simulink model "AMR_MotorStartupUnit_MoboticDrive_24a"  (R2024a)
settings: configuration reference "SharedConfig" (kept outside this file)
settings Model: DataDictionary=configuration_dictionary.sldd  SimulationMode=external  Creator=matlab.cut  LastModifiedBy=rodri
settings ConfigSetRef: SourceName=SharedConfig

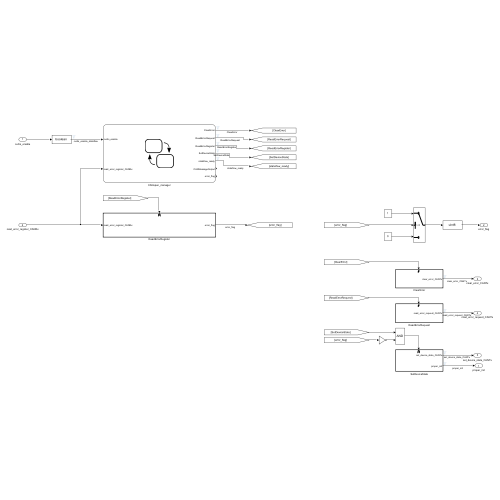
[thumbnail: Simulink's stored preview of the top-level diagram]
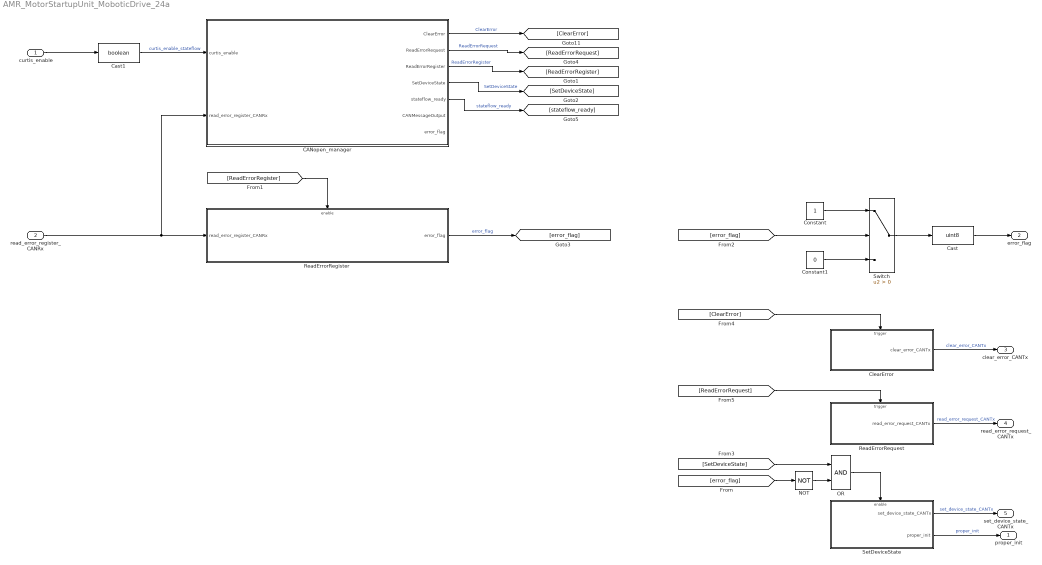
== system AMR_MotorStartupUnit_MoboticDrive_24a ==
  curtis_enable : Inport
  read_error_register_CANRx : Inport  Port=2
  CANopen_manager : Stateflow chart  TreatAsAtomicUnit=on
  Cast : DataTypeConversion  OutDataTypeStr=uint8  SaturateOnIntegerOverflow=off  RndMeth=Floor
  Cast1 : DataTypeConversion  OutDataTypeStr=boolean  SaturateOnIntegerOverflow=off  RndMeth=Floor
  ClearError : Subsystem  TreatAsAtomicUnit=on
  Constant : Constant
  Constant1 : Constant  Value=0
  NOT : Logic  Operator=NOT  IconShape=distinctive  AllPortsSameDT=off  OutDataTypeStr=boolean
  OR : Logic  AllPortsSameDT=off  OutDataTypeStr=boolean
  ReadErrorRegister : Subsystem  TreatAsAtomicUnit=on
  ReadErrorRequest : Subsystem  TreatAsAtomicUnit=on
  SetDeviceState : Subsystem  TreatAsAtomicUnit=on
  Switch : Switch  Criteria=u2 > Threshold  SaturateOnIntegerOverflow=off  InputSameDT=off
  proper_init : Outport
  error_flag : Outport  Port=2
  clear_error_CANTx : Outport  Port=3
  read_error_request_CANTx : Outport  Port=4
  set_device_state_CANTx : Outport  Port=5
  wires:
  [error_flag] -> Switch/2
  Switch/1 -> Cast/1
  Cast/1 -> error_flag/1
  [SetDeviceState] -> OR/1
  [error_flag] -> NOT/1
  curtis_enable/1 -> Cast1/1
  Constant/1 -> Switch/1
  Constant1/1 -> Switch/3
  ReadErrorRegister/1(error_flag) -> [error_flag]  "error_flag"
  NOT/1 -> OR/2
  [ReadErrorRegister] -> ReadErrorRegister/Enable
  ClearError/1(clear_error_CANTx) -> clear_error_CANTx/1  "clear_error_CANTx"
  read_error_register_CANRx/1 -> CANopen_manager/2(read_error_register_CANRx), ReadErrorRegister/1(read_error_register_CANRx)
  SetDeviceState/1(set_device_state_CANTx) -> set_device_state_CANTx/1  "set_device_state_CANTx"
  ReadErrorRequest/1(read_error_request_CANTx) -> read_error_request_CANTx/1  "read_error_request_CANTx"
  SetDeviceState/2(proper_init) -> proper_init/1  "proper_init"
  CANopen_manager/2(ReadErrorRequest) -> [ReadErrorRequest]  "ReadErrorRequest"
  CANopen_manager/5(stateflow_ready) -> [stateflow_ready]  "stateflow_ready"
  Cast1/1 -> CANopen_manager/1(curtis_enable)  "curtis_enable_stateflow"
  CANopen_manager/3(ReadErrorRegister) -> [ReadErrorRegister]  "ReadErrorRegister"
  CANopen_manager/1(ClearError) -> [ClearError]  "ClearError"
  CANopen_manager/4(SetDeviceState) -> [SetDeviceState]  "SetDeviceState"
  OR/1 -> SetDeviceState/Enable
  [ClearError] -> ClearError/Trigger
  [ReadErrorRequest] -> ReadErrorRequest/Trigger

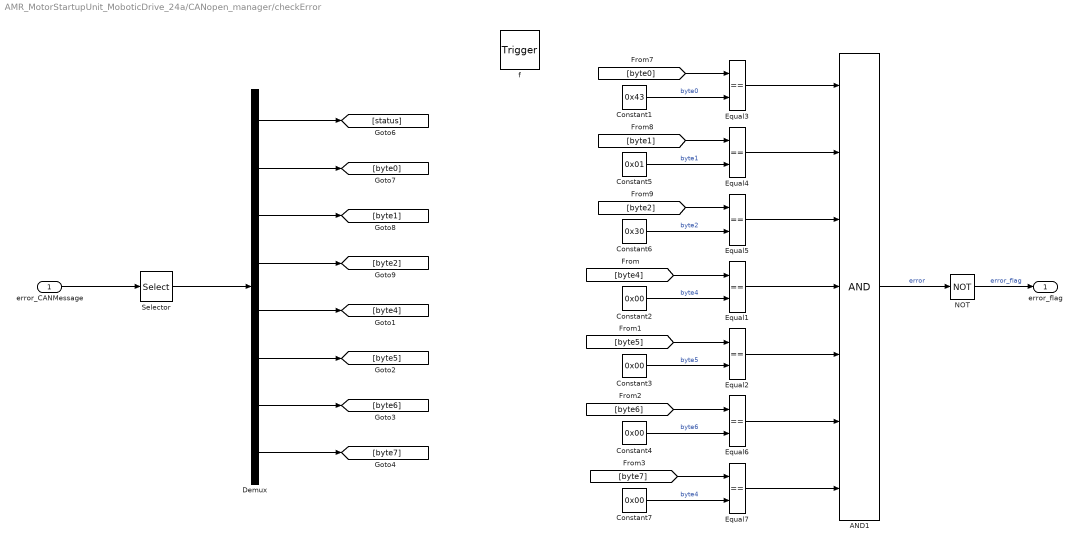
== system AMR_MotorStartupUnit_MoboticDrive_24a/CANopen_manager/checkError ==
  error_CANMessage : Inport  OutDataTypeStr=double  PortDimensions=1
  f : TriggerPort  TriggerType=function-call  VariantControl=(inherit)
      settings: CopyFcn=Stateflow.SLINSF.SimulinkMan.removeBlockPreDeleteFcn  PreDeleteFcn=Stateflow.SLINSF.SimulinkMan.unsafePredeleteFcn
  AND1 : Logic  Inputs=7  AllPortsSameDT=off  OutDataTypeStr=boolean
  Constant1 : Constant  Value=0x43
  Constant{2..4,7} (4 alike) : Constant  Value=0x00
  Constant5 : Constant  Value=0x01
  Constant6 : Constant  Value=0x30
  Demux : Demux  Outputs=8
  Equal{1..7} (7 alike) : RelationalOperator  Operator===  OutDataTypeStr=boolean  RndMeth=Simplest  InputSameDT=off
  NOT : Logic  Operator=NOT  IconShape=distinctive  AllPortsSameDT=off  OutDataTypeStr=boolean
  Selector : Selector  IndexMode=Zero-based  InputPortWidth=9  IndexOptions=Index vector (dialog)  Indices=[0:3,5:8]  OutputSizes=1
  error_flag : Outport
  wires:
  [byte5] -> Equal2/1
  Demux/1 -> [status]
  Demux/8 -> [byte7]
  [byte2] -> Equal5/1
  Constant7/1 -> Equal7/2  "byte4"
  Constant3/1 -> Equal2/2  "byte5"
  Equal3/1 -> AND1/1
  [byte6] -> Equal6/1
  Constant2/1 -> Equal1/2  "byte4"
  Constant5/1 -> Equal4/2  "byte1"
  Constant1/1 -> Equal3/2  "byte0"
  Demux/3 -> [byte1]
  Demux/4 -> [byte2]
  Demux/7 -> [byte6]
  [byte4] -> Equal1/1
  [byte7] -> Equal7/1
  Equal4/1 -> AND1/2
  Equal5/1 -> AND1/3
  Demux/5 -> [byte4]
  error_CANMessage/1 -> Selector/1
  Demux/2 -> [byte0]
  Demux/6 -> [byte5]
  Selector/1 -> Demux/1
  Equal7/1 -> AND1/7
  Constant6/1 -> Equal5/2  "byte2"
  Equal1/1 -> AND1/4
  Equal6/1 -> AND1/6
  AND1/1 -> NOT/1  "error"
  [byte1] -> Equal4/1
  Equal2/1 -> AND1/5
  Constant4/1 -> Equal6/2  "byte6"
  [byte0] -> Equal3/1
  NOT/1 -> error_flag/1  "error_flag"

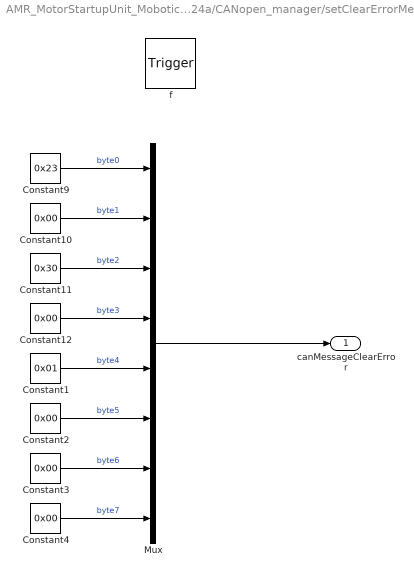
== system AMR_MotorStartupUnit_MoboticDrive_24a/CANopen_manager/setClearErrorMessage ==
  f : TriggerPort  TriggerType=function-call  VariantControl=(inherit)
      settings: CopyFcn=Stateflow.SLINSF.SimulinkMan.removeBlockPreDeleteFcn  PreDeleteFcn=Stateflow.SLINSF.SimulinkMan.unsafePredeleteFcn
  Constant1 : Constant  Value=0x01
  Constant{2..4,10,12} (5 alike) : Constant  Value=0x00
  Constant11 : Constant  Value=0x30
  Constant9 : Constant  Value=0x23
  Mux : Mux  Inputs=8
  canMessageClearError : Outport
  wires:
  Constant10/1 -> Mux/2  "byte1"
  Constant3/1 -> Mux/7  "byte6"
  Constant12/1 -> Mux/4  "byte3"
  Constant4/1 -> Mux/8  "byte7"
  Constant1/1 -> Mux/5  "byte4"
  Mux/1 -> canMessageClearError/1
  Constant11/1 -> Mux/3  "byte2"
  Constant9/1 -> Mux/1  "byte0"
  Constant2/1 -> Mux/6  "byte5"

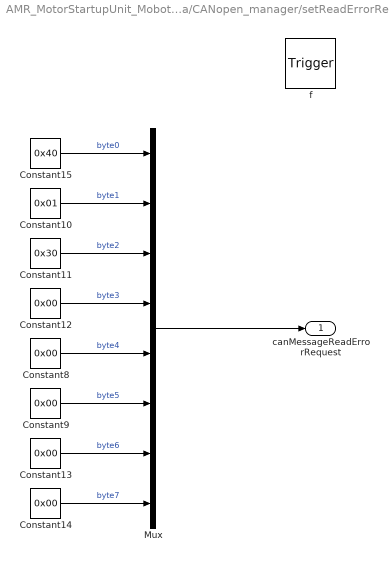
== system AMR_MotorStartupUnit_MoboticDrive_24a/CANopen_manager/setReadErrorRequest ==
  f : TriggerPort  TriggerType=function-call  VariantControl=(inherit)
      settings: CopyFcn=Stateflow.SLINSF.SimulinkMan.removeBlockPreDeleteFcn  PreDeleteFcn=Stateflow.SLINSF.SimulinkMan.unsafePredeleteFcn
  Constant10 : Constant  Value=0x01
  Constant11 : Constant  Value=0x30
  Constant{8..9,12..14} (5 alike) : Constant  Value=0x00
  Constant15 : Constant  Value=0x40
  Mux : Mux  Inputs=8
  canMessageReadErrorRequest : Outport
  wires:
  Constant13/1 -> Mux/7  "byte6"
  Constant9/1 -> Mux/6  "byte5"
  Constant8/1 -> Mux/5  "byte4"
  Constant12/1 -> Mux/4  "byte3"
  Constant10/1 -> Mux/2  "byte1"
  Constant15/1 -> Mux/1  "byte0"
  Constant11/1 -> Mux/3  "byte2"
  Constant14/1 -> Mux/8  "byte7"
  Mux/1 -> canMessageReadErrorRequest/1

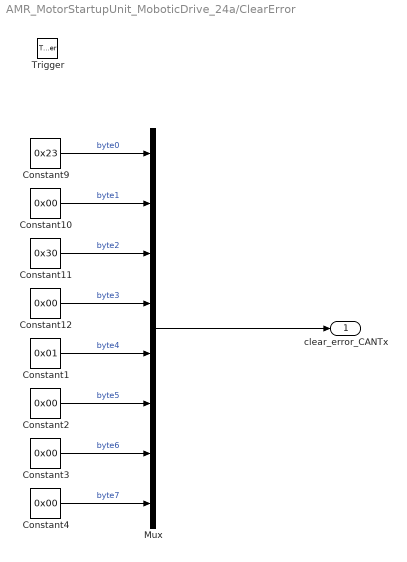
== system AMR_MotorStartupUnit_MoboticDrive_24a/ClearError ==
  Trigger : TriggerPort  VariantControl=(inherit)  PortDimensions=1
  Constant1 : Constant  Value=0x01
  Constant{2..4,10,12} (5 alike) : Constant  Value=0x00
  Constant11 : Constant  Value=0x30
  Constant9 : Constant  Value=0x23
  Mux : Mux  Inputs=8
  clear_error_CANTx : Outport  OutputWhenDisabled=reset  InitialOutput=0
  wires:
  Mux/1 -> clear_error_CANTx/1
  Constant4/1 -> Mux/8  "byte7"
  Constant9/1 -> Mux/1  "byte0"
  Constant10/1 -> Mux/2  "byte1"
  Constant11/1 -> Mux/3  "byte2"
  Constant12/1 -> Mux/4  "byte3"
  Constant1/1 -> Mux/5  "byte4"
  Constant2/1 -> Mux/6  "byte5"
  Constant3/1 -> Mux/7  "byte6"

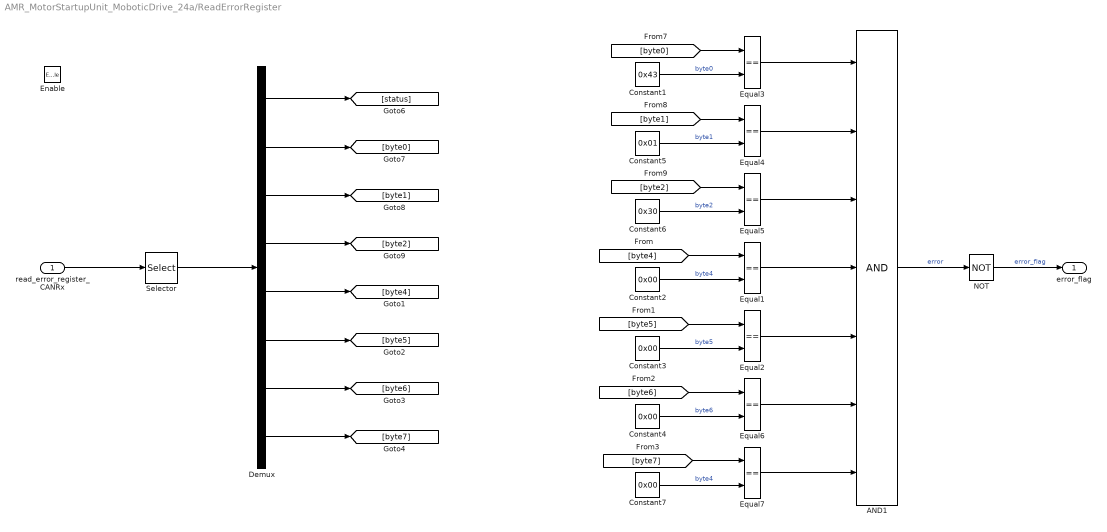
== system AMR_MotorStartupUnit_MoboticDrive_24a/ReadErrorRegister ==
  read_error_register_CANRx : Inport
  Enable : EnablePort  StatesWhenEnabling=reset
  AND1 : Logic  Inputs=7  AllPortsSameDT=off  OutDataTypeStr=boolean
  Constant1 : Constant  Value=0x43
  Constant{2..4,7} (4 alike) : Constant  Value=0x00
  Constant5 : Constant  Value=0x01
  Constant6 : Constant  Value=0x30
  Demux : Demux  Outputs=8
  Equal{1..7} (7 alike) : RelationalOperator  Operator===  OutDataTypeStr=boolean  RndMeth=Simplest  InputSameDT=off
  NOT : Logic  Operator=NOT  IconShape=distinctive  AllPortsSameDT=off  OutDataTypeStr=boolean
  Selector : Selector  IndexMode=Zero-based  InputPortWidth=9  IndexOptions=Index vector (dialog)  Indices=[0:3,5:8]  OutputSizes=1
  error_flag : Outport  InitialOutput=[0]
  wires:
  [byte0] -> Equal3/1
  Constant5/1 -> Equal4/2  "byte1"
  [byte1] -> Equal4/1
  [byte2] -> Equal5/1
  Demux/8 -> [byte7]
  Demux/4 -> [byte2]
  Demux/2 -> [byte0]
  Demux/1 -> [status]
  Demux/7 -> [byte6]
  Demux/6 -> [byte5]
  read_error_register_CANRx/1 -> Selector/1
  Demux/5 -> [byte4]
  Constant6/1 -> Equal5/2  "byte2"
  Demux/3 -> [byte1]
  Constant1/1 -> Equal3/2  "byte0"
  Constant2/1 -> Equal1/2  "byte4"
  [byte4] -> Equal1/1
  [byte5] -> Equal2/1
  Constant3/1 -> Equal2/2  "byte5"
  Constant4/1 -> Equal6/2  "byte6"
  [byte6] -> Equal6/1
  [byte7] -> Equal7/1
  Constant7/1 -> Equal7/2  "byte4"
  AND1/1 -> NOT/1  "error"
  NOT/1 -> error_flag/1  "error_flag"
  Equal3/1 -> AND1/1
  Equal4/1 -> AND1/2
  Equal5/1 -> AND1/3
  Equal1/1 -> AND1/4
  Equal2/1 -> AND1/5
  Equal6/1 -> AND1/6
  Equal7/1 -> AND1/7
  Selector/1 -> Demux/1

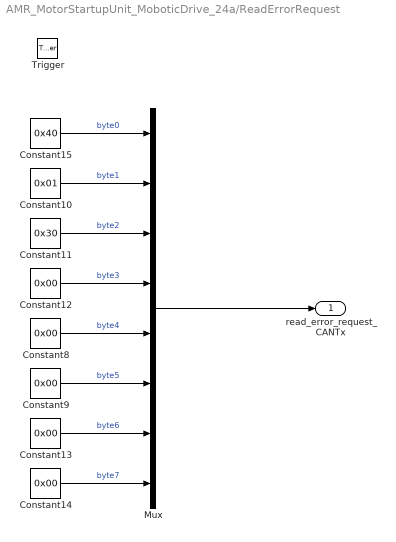
== system AMR_MotorStartupUnit_MoboticDrive_24a/ReadErrorRequest ==
  Trigger : TriggerPort  VariantControl=(inherit)  PortDimensions=1
  Constant10 : Constant  Value=0x01
  Constant11 : Constant  Value=0x30
  Constant{8..9,12..14} (5 alike) : Constant  Value=0x00
  Constant15 : Constant  Value=0x40
  Mux : Mux  Inputs=8
  read_error_request_CANTx : Outport  OutputWhenDisabled=reset  InitialOutput=0
  wires:
  Constant11/1 -> Mux/3  "byte2"
  Constant9/1 -> Mux/6  "byte5"
  Constant14/1 -> Mux/8  "byte7"
  Constant15/1 -> Mux/1  "byte0"
  Mux/1 -> read_error_request_CANTx/1
  Constant10/1 -> Mux/2  "byte1"
  Constant12/1 -> Mux/4  "byte3"
  Constant8/1 -> Mux/5  "byte4"
  Constant13/1 -> Mux/7  "byte6"

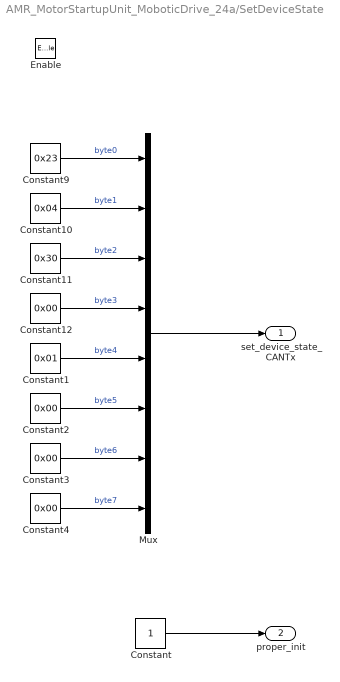
== system AMR_MotorStartupUnit_MoboticDrive_24a/SetDeviceState ==
  Enable : EnablePort
  Constant : Constant
  Constant1 : Constant  Value=0x01
  Constant10 : Constant  Value=0x04
  Constant11 : Constant  Value=0x30
  Constant{2..4,12} (4 alike) : Constant  Value=0x00
  Constant9 : Constant  Value=0x23
  Mux : Mux  Inputs=8
  set_device_state_CANTx : Outport  OutputWhenDisabled=reset  InitialOutput=0
  proper_init : Outport  Port=2  OutputWhenDisabled=reset  InitialOutput=0
  wires:
  Constant10/1 -> Mux/2  "byte1"
  Constant4/1 -> Mux/8  "byte7"
  Constant12/1 -> Mux/4  "byte3"
  Constant9/1 -> Mux/1  "byte0"
  Constant1/1 -> Mux/5  "byte4"
  Constant2/1 -> Mux/6  "byte5"
  Constant3/1 -> Mux/7  "byte6"
  Constant11/1 -> Mux/3  "byte2"
  Mux/1 -> set_device_state_CANTx/1
  Constant/1 -> proper_init/1

== stateflow chart AMR_MotorStartupUnit_MoboticDrive_24a/CANopen_manager ==
  state SetDeviceStateON
    entry:
    ClearError = 0; % send clear error command
    ReadErrorRegister = 0;
    ReadErrorRegister = 0;
    SetDeviceState = 1;
    stateflow_ready = 0;
    exit:
    SetDeviceState = 0;
  state idle
    entry:
    ClearError = 0; % send clear error command
    ReadErrorRequest = 0; % request to read error
    ReadErrorRegister = 0; % read error register
    SetDeviceState = 0; % send enable command
  state error_flag = checkError(error_CANMessage) [function]
  state ReadErrorRegister
    entry:
    ClearError = 0;
    ReadErrorRequest = 0;
    error_flag = checkError(read_error_register_CANRx);
    SetDeviceState = 0;
    stateflow_ready = 0;
  state wait_for_curtis
    entry:
    ClearError = 0; % send clear error command
    ReadErrorRequest = 0; % request to read error
    ReadErrorRegister = 0; % read error register
    SetDeviceState = 0; % send enable command
    exit:
    i = i+1;
  state canMessageClearError = setClearErrorMessage [function]
  state canMessageReadErrorRequest = setReadErrorRequest [function]
  state ClearError
    entry:
    CANMessageOutput = setClearErrorMessage();
    ReadErrorRequest = 0;
    ReadErrorRegister = 0;
    SetDeviceState = 0;
    stateflow_ready = 0;
    exit:
    ClearError = 0;
  state ReadErrorRequest
    entry:
    ClearError = 0;
    CANMessageOutput = setReadErrorRequest();
    ReadErrorRegister = 0;
    SetDeviceState = 0;
    stateflow_ready = 0;
    exit:
    ReadErrorRequest = 0;
  (default) -> idle : {i = 5; stateflow_ready = 0}
  idle -> idle [order 2]
  SetDeviceStateON -> idle : [after(50,msec)]
      | {stateflow_ready = 1}
  idle -> wait_for_curtis [order 1] : [curtis_enable == true]
      | {i = 0; stateflow_ready = 0;}
  ReadErrorRegister -> SetDeviceStateON [order 1] : after(50,msec)
      | [i  == 3]
      | {ReadErrorRegister = 0}
  ReadErrorRegister -> wait_for_curtis [order 2] : after(50,msec)
      | [i < 3]
  wait_for_curtis -> ClearError : after(500,msec)
  ReadErrorRequest -> ReadErrorRegister : after(50,msec)
  ClearError -> ReadErrorRequest : after(50,msec)
  data: error_flag function_output; error_CANMessage function_input double size=1; canMessageClearError function_output; canMessageReadErrorRequest function_output; curtis_enable input; ClearError output; ReadErrorRequest output; ReadErrorRegister output; SetDeviceState output; stateflow_ready output; i local; CANMessageOutput output; error_flag output; read_error_register_CANRx input
